simulink model "PD_controller"  (R2019b)
settings: Solver=ode4  StartTime=0.0  StopTime=100  FixedStep=0.01  RelTol=1e-3
settings Model: Creator=USER  LastModifiedBy=USER

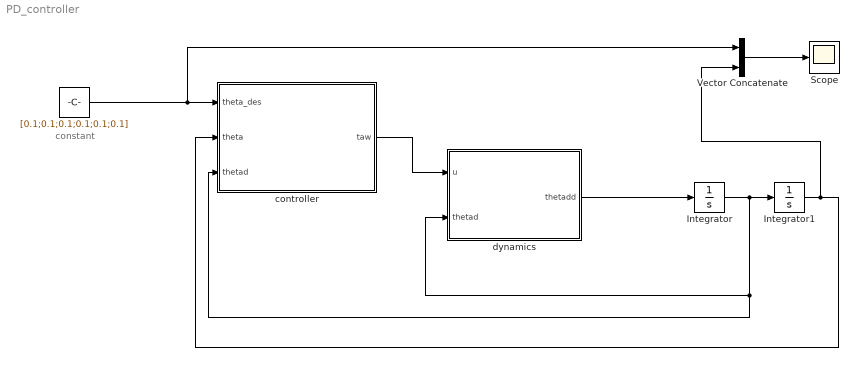
== system PD_controller ==
  note: constant
  " " : Constant  Value=[0.1;0.1;0.1;0.1;0.1;0.1]
  Integrator : Integrator  InitialCondition=[0.1;0.1;0.1;0.1;0.1;0.1]
  Integrator1 : Integrator  InitialCondition=[0.1;0.1;0.1;0.1;0.1;0.1]
  Scope : Scope
  Vector Concatenate : Concatenate
  controller : MATLAB Function  TreatAsAtomicUnit=on
  dynamics : MATLAB Function  TreatAsAtomicUnit=on
  wires:
  dynamics/1(thetadd) -> Integrator/1
  Integrator/1 -> dynamics/2(thetad), controller/3(thetad), Integrator1/1
  Integrator1/1 -> Vector Concatenate/2, controller/2(theta)
  controller/1(taw) -> dynamics/1(u)
  Vector Concatenate/1 -> Scope/1
  " "/1 -> Vector Concatenate/1, controller/1(theta_des)

== matlab function PD_controller/controller ==
  data: taw output; theta_des input; theta input; thetad input
function taw = fcn(theta_des,theta,thetad)
G=[                125/576460752303423488;
        6243369967885135/2199023255552;
        1843278687284175/4398046511104;
 -7769952016327311/1152921504606846976;
     2257351121598699/2251799813685248;
                                     1];
M=[ 52.4722   -0.0003    0.0028   -0.0503   -0.0001    0.0000;
  104.8982  290.5285  163.8569   85.7264   85.2726   85.2667;
   85.2667  115.8130  148.4693   85.6721   85.2726   85.2667;
   -0.0119   -0.0070   -0.0097   -0.0017   -0.0067   -0.0067;
    0.6575    0.7170    0.9633    0.6800    0.6687    0.6627;
         1         1         1         1         1         1]
C=[261.8493         0         0   -0.0005         0         0;
   -4.1701   76.1836   58.8031    0.3261   -0.0000   -0.0000;
  -60.4552   -6.5177    2.5168    0.0520    0.0000    0.0000;
   -0.0055         0         0    0.0005         0         0;
   -0.4221   -0.0217   -0.0460   -0.3403         0         0;
         1         1         1         1         1         1]

e=theta_des-theta
edot=-thetad
Kp=[1 0 0 0 0 0;0 1 0 0 0 0;0 0 1 0 0 0;0 0 0 1 0 0;0 0 0 0 1 0;0 0 0 0 0 1]
Kd=[.1 0 0 0 0 0;0 .1 0 0 0 0;0 0 .1 0 0 0;0 0 0 .1 0 0;0 0 0 0 .1 0;0 0 0 0 0 .1]
taw=Kd*edot+Kp*e

== matlab function PD_controller/dynamics ==
  data: u input; thetadd output; thetad input
function thetadd = fcn(u,thetad)
G=[                125/576460752303423488;
        6243369967885135/2199023255552;
        1843278687284175/4398046511104;
 -7769952016327311/1152921504606846976;
     2257351121598699/2251799813685248;
                                    1];
M=[ 52.4722   -0.0003    0.0028   -0.0503   -0.0001    0.0000;
  104.8982  290.5285  163.8569   85.7264   85.2726   85.2667;
   85.2667  115.8130  148.4693   85.6721   85.2726   85.2667;
   -0.0119   -0.0070   -0.0097   -0.0017   -0.0067   -0.0067;
    0.6575    0.7170    0.9633    0.6800    0.6687    0.6627;
         1         1         1         1         1         1]
C=[261.8493         0         0   -0.0005         0         0;
   -4.1701   76.1836   58.8031    0.3261   -0.0000   -0.0000;
  -60.4552   -6.5177    2.5168    0.0520    0.0000    0.0000;
   -0.0055         0         0    0.0005         0         0;
   -0.4221   -0.0217   -0.0460   -0.3403         0         0;
         1         1         1         1         1        1]
     thetadd=inv(M)*(u-C*thetad-G);
